simulink model "CDMA"  (Simulink 7.6)
settings: Solver=ode45  StartTime=0.0  StopTime=30  RelTol=1e-3
libraries: commrandsrc2 x3, dsparch4 x3, simulink x2, commchan3 x1, commseqgen2 x1
settings Model: Creator=matlab  LastModifiedBy=matlab

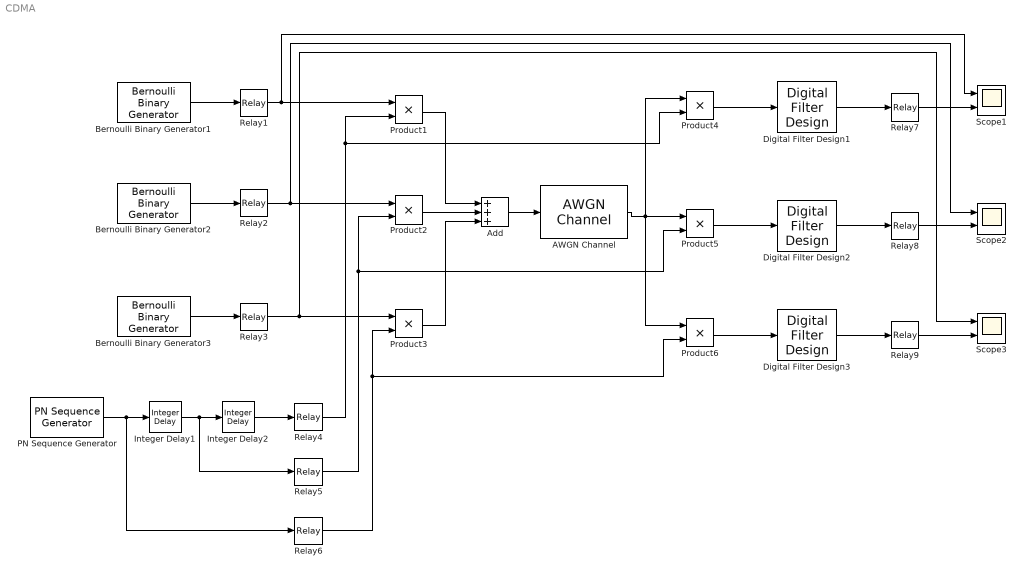
== system CDMA ==
  AWGN Channel : commchan3/AWGN Channel  SystemSampleTime=-1  InputProcessing=Columns as channels (frame based)  seed=67  noiseMode=Variance from mask  EbNodB=10  EsNodB=10  SNRdB=10  bitsPerSym=1  Ps=1  Tsym=1  variance=0.01
  Add : Sum  Inputs=+++
  Bernoulli Binary Generator1 : commrandsrc2/Bernoulli Binary Generator  DialogController=commDDGCreate  DialogControllerArgs=DataTag1  SystemSampleTime=-1  P=0.5  seed=51  Ts=1  frameBased=off  sampPerFrame=1  orient=off  outDataType=double
  Bernoulli Binary Generator2 : commrandsrc2/Bernoulli Binary Generator  DialogController=commDDGCreate  DialogControllerArgs=DataTag2  SystemSampleTime=-1  P=0.5  seed=61  Ts=1  frameBased=off  sampPerFrame=1  orient=off  outDataType=double
  Bernoulli Binary Generator3 : commrandsrc2/Bernoulli Binary Generator  DialogController=commDDGCreate  DialogControllerArgs=DataTag3  SystemSampleTime=-1  P=0.5  seed=71  Ts=1  frameBased=off  sampPerFrame=1  orient=off  outDataType=double
  Digital Filter Design1 : dsparch4/Digital Filter Design  SystemSampleTime=-1  mwdsp_browser_bugfix_var=off
      link override Digital Filter: TypePopup=FIR (all zeros)  FIRFiltStruct=Direct form  NumCoeffs=[3.82142455213508e-005 -0.000119915251257174 -0.000306564799154108 -0.000644314291099943 -0.0011600436778058 -0.00187212162025008 -0.00277549514382723 -0.00383217796983655 -0.00496558749977943 -0.00606042632172775 -0.00696916062638655 -0.00752634267391555 -0.00756950840880499 -0.00696556087151318 -0.00563846070575491 -0.00359502771755077 -0.000943233435757262 0.00210111832774632 0.005222787307113 0.00803275326341323 0.0101097591791879 0.0110547445773942 0.0105525399874693 0.00843231647788946 0.00471821217894827 -0.000338851631946369 -0.00625525061747478 -0.0123390374896814 -0.0177456212686449 -0.0215606778407806 -0.022902471178421 -0.021031980406395 -0.0154578052507362 -0.00602127930236947 0.00705115252524928 0.0231361290739701 0.0412476590327594 0.0601166629618959 0.0783058723421673 0.0943519541397477 0.106914513777345 0.114917842765444 0.117665849116606 0.114917842765444 0.106914513777345 0.0943519541397477 0.0783058723421673 0.0601166629618959 0.0412476590327594 0.0231361290739701 0.00705115252524928 -0.00602127930236947 -0.0154578052507362 -0.021031980406395 -0.022902471178421 -0.0215606778407806 -0.0177456212686449 -0.0123390374896814 -0.00625525061747478 -0.000338851631946369 0.00471821217894827 0.00843231647788946 0.0105525399874693 0.0110547445773942 0.0101097591791879 0.00803275326341323 0.005222787307113 0.00210111832774632 -0.000943233435757262 -0.00359502771755077 -0.00563846070575491 -0.00696556087151318 -0.00756950840880499 -0.00752634267391555 -0.00696916062638655 -0.00606042632172775 -0.00496558749977943 -0.00383217796983655 -0.00277549514382723 -0.00187212162025008 -0.0011600436778058 -0.000644314291099943 -0.000306564799154108 -0.000119915251257174 3.82142455213508e-005]
  Digital Filter Design2 : dsparch4/Digital Filter Design  SystemSampleTime=-1  mwdsp_browser_bugfix_var=off
      link override Digital Filter: TypePopup=FIR (all zeros)  FIRFiltStruct=Direct form  NumCoeffs=[3.82142455213508e-005 -0.000119915251257174 -0.000306564799154108 -0.000644314291099943 -0.0011600436778058 -0.00187212162025008 -0.00277549514382723 -0.00383217796983655 -0.00496558749977943 -0.00606042632172775 -0.00696916062638655 -0.00752634267391555 -0.00756950840880499 -0.00696556087151318 -0.00563846070575491 -0.00359502771755077 -0.000943233435757262 0.00210111832774632 0.005222787307113 0.00803275326341323 0.0101097591791879 0.0110547445773942 0.0105525399874693 0.00843231647788946 0.00471821217894827 -0.000338851631946369 -0.00625525061747478 -0.0123390374896814 -0.0177456212686449 -0.0215606778407806 -0.022902471178421 -0.021031980406395 -0.0154578052507362 -0.00602127930236947 0.00705115252524928 0.0231361290739701 0.0412476590327594 0.0601166629618959 0.0783058723421673 0.0943519541397477 0.106914513777345 0.114917842765444 0.117665849116606 0.114917842765444 0.106914513777345 0.0943519541397477 0.0783058723421673 0.0601166629618959 0.0412476590327594 0.0231361290739701 0.00705115252524928 -0.00602127930236947 -0.0154578052507362 -0.021031980406395 -0.022902471178421 -0.0215606778407806 -0.0177456212686449 -0.0123390374896814 -0.00625525061747478 -0.000338851631946369 0.00471821217894827 0.00843231647788946 0.0105525399874693 0.0110547445773942 0.0101097591791879 0.00803275326341323 0.005222787307113 0.00210111832774632 -0.000943233435757262 -0.00359502771755077 -0.00563846070575491 -0.00696556087151318 -0.00756950840880499 -0.00752634267391555 -0.00696916062638655 -0.00606042632172775 -0.00496558749977943 -0.00383217796983655 -0.00277549514382723 -0.00187212162025008 -0.0011600436778058 -0.000644314291099943 -0.000306564799154108 -0.000119915251257174 3.82142455213508e-005]
  Digital Filter Design3 : dsparch4/Digital Filter Design  SystemSampleTime=-1  mwdsp_browser_bugfix_var=off
      link override Digital Filter: TypePopup=FIR (all zeros)  FIRFiltStruct=Direct form  NumCoeffs=[3.82142455213508e-005 -0.000119915251257174 -0.000306564799154108 -0.000644314291099943 -0.0011600436778058 -0.00187212162025008 -0.00277549514382723 -0.00383217796983655 -0.00496558749977943 -0.00606042632172775 -0.00696916062638655 -0.00752634267391555 -0.00756950840880499 -0.00696556087151318 -0.00563846070575491 -0.00359502771755077 -0.000943233435757262 0.00210111832774632 0.005222787307113 0.00803275326341323 0.0101097591791879 0.0110547445773942 0.0105525399874693 0.00843231647788946 0.00471821217894827 -0.000338851631946369 -0.00625525061747478 -0.0123390374896814 -0.0177456212686449 -0.0215606778407806 -0.022902471178421 -0.021031980406395 -0.0154578052507362 -0.00602127930236947 0.00705115252524928 0.0231361290739701 0.0412476590327594 0.0601166629618959 0.0783058723421673 0.0943519541397477 0.106914513777345 0.114917842765444 0.117665849116606 0.114917842765444 0.106914513777345 0.0943519541397477 0.0783058723421673 0.0601166629618959 0.0412476590327594 0.0231361290739701 0.00705115252524928 -0.00602127930236947 -0.0154578052507362 -0.021031980406395 -0.022902471178421 -0.0215606778407806 -0.0177456212686449 -0.0123390374896814 -0.00625525061747478 -0.000338851631946369 0.00471821217894827 0.00843231647788946 0.0105525399874693 0.0110547445773942 0.0101097591791879 0.00803275326341323 0.005222787307113 0.00210111832774632 -0.000943233435757262 -0.00359502771755077 -0.00563846070575491 -0.00696556087151318 -0.00756950840880499 -0.00752634267391555 -0.00696916062638655 -0.00606042632172775 -0.00496558749977943 -0.00383217796983655 -0.00277549514382723 -0.00187212162025008 -0.0011600436778058 -0.000644314291099943 -0.000306564799154108 -0.000119915251257174 3.82142455213508e-005]
  Integer Delay1 : simulink/Discrete/Integer Delay  NumDelays=4  vinit=0.0  samptime=-1
  Integer Delay2 : simulink/Discrete/Integer Delay  NumDelays=3  vinit=0.0  samptime=-1
  PN Sequence Generator : commseqgen2/PN Sequence Generator  poly=[1 0 0 0 0 1 1]  ini_sta=[0 0 0 0 0 1]  outBitMaskSource=Dialog parameter  shift=0  Ts=0.01  frameBased=off  sampPerFrame=1  reset=off  bitPackedOutputs=off  outDataType=double  numPackedBits=8  bitPackDataSigned=off  bitPackedOutDType=double
  Product{1..6} (6 alike) : Product  RndMeth=Zero
  Relay{1..6} (6 alike) : Relay  OnSwitchValue=0.9  OffSwitchValue=0.1  OffOutputValue=-1  SampleTime=0.01
  Relay7 : Relay  OnSwitchValue=0.5  OffSwitchValue=-0.5  OffOutputValue=-1  SampleTime=0.01
  Relay8 : Relay  OnSwitchValue=0.5  OffSwitchValue=-0.5  OffOutputValue=-1
  Relay9 : Relay  OnSwitchValue=0.5  OffSwitchValue=-0.5  OffOutputValue=-1  SampleTime=0.01
  Scope1 : Scope  NumInputPorts=2
      settings: YMin=-5~-5  YMax=5~5
  Scope2 : Scope  NumInputPorts=2
      settings: YMin=-5~-5  YMax=5~5
  Scope3 : Scope  NumInputPorts=2
      settings: YMin=-5~-5  YMax=5~5  SaveName=ScopeData2
  wires:
  Bernoulli Binary Generator1/1 -> Relay1/1
  Bernoulli Binary Generator2/1 -> Relay2/1
  Bernoulli Binary Generator3/1 -> Relay3/1
  Relay1/1 -> Product1/1, Scope1/1
  PN Sequence Generator/1 -> Integer Delay1/1, Relay6/1
  Integer Delay1/1 -> Integer Delay2/1, Relay5/1
  Integer Delay2/1 -> Relay4/1
  Relay4/1 -> Product1/2, Product4/2
  Relay2/1 -> Product2/1, Scope2/1
  Relay3/1 -> Product3/1, Scope3/1
  Relay5/1 -> Product2/2, Product5/2
  Relay6/1 -> Product3/2, Product6/2
  Product2/1 -> Add/2
  Product1/1 -> Add/1
  Product3/1 -> Add/3
  Add/1 -> AWGN Channel/1
  AWGN Channel/1 -> Product5/1, Product4/1, Product6/1
  Product4/1 -> Digital Filter Design1/1
  Product5/1 -> Digital Filter Design2/1
  Product6/1 -> Digital Filter Design3/1
  Digital Filter Design1/1 -> Relay7/1
  Digital Filter Design2/1 -> Relay8/1
  Digital Filter Design3/1 -> Relay9/1
  Relay7/1 -> Scope1/2
  Relay8/1 -> Scope2/2
  Relay9/1 -> Scope3/2
